simulink model "environment_model_task3"  (Simulink 8.8)
settings: Solver=ode45  StartTime=0.0  StopTime=20000  MaxStep=1  RelTol=1e-3  AbsTol=1e-6  EnableMultiTasking=on
values from neighbouring files (symbols this model uses):
  c = input(5)    [QuatController.m]    (also in main.m = C_optimal; task3b.m = copt)
  k = input(4)    [QuatController.m]    (also in main.m = K_optimal; task3b.m = kopt)
undefined symbols (not defined in the file or in its folder): initial_r, initial_v
settings Model: SuppressorTable=22 serialization::archive 11 0 3 0 0 0 0 0  Creator=menjkim  LastModifiedBy=jamesthomson
settings DataIOCC: SignalLoggingSaveFormat=Dataset  InspectSignalLogs=on
settings OptimizationCC: ExpressionDepthLimit=2147483647
settings DebuggingCC: SolverPrmCheckMsg=warning  FcnCallInpInsideContextMsg=error
settings GRTTargetCC: CombineOutputUpdateFcns=on  GRTInterface=off

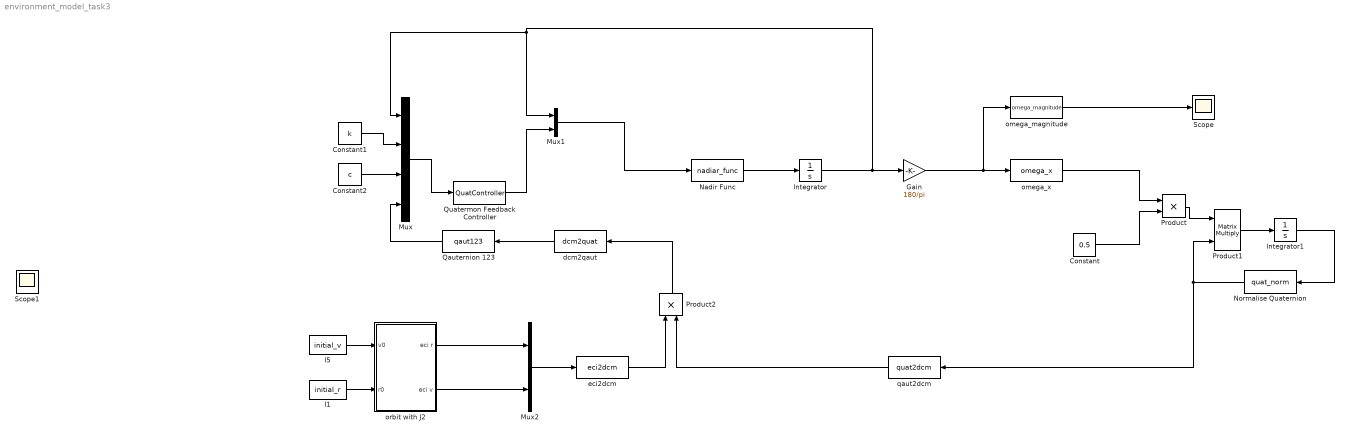
== system environment_model_task3 ==
  Constant : Constant  Value=0.5
  Constant1 : Constant  Value=k
  Constant2 : Constant  Value=c
  Gain : Gain  Gain=180/pi
  I1 : Constant  Value=initial_r
  I5 : Constant  Value=initial_v
  Integrator : Integrator  InitialCondition=[-0.1; 0.1; -0.2]
  Integrator1 : Integrator  InitialCondition=[0.1754; 0.5951; -0.7329; 0.2798]
  Mux : Mux
  Mux1 : Mux  Inputs=2
  Mux2 : Mux  Inputs=2
  Nadir Func : MATLABFcn  MATLABFcn=nadiar_func
  Normalise Quaternion : MATLABFcn  MATLABFcn=quat_norm  Output1D=off
  Product : Product
  Product1 : Product  Multiplication=Matrix(*)
  Product2 : Product
  Qauternion 123 : MATLABFcn  MATLABFcn=qaut123  Output1D=off
  Quatermon Feedback Controller : MATLABFcn  MATLABFcn=QuatController  Output1D=off
  Scope : Scope
  dcm2qaut : MATLABFcn  MATLABFcn=dcm2quat
  eci2dcm : MATLABFcn  MATLABFcn=eci2dcm  Output1D=off
  omega_magnitude : MATLABFcn  MATLABFcn=omega_magnitude
  omega_x : MATLABFcn  MATLABFcn=omega_x  Output1D=off
  orbit with J2 : Subsystem
  qaut2dcm : MATLABFcn  MATLABFcn=quat2dcm  Output1D=off
  Scope1 : Scope
  wires:
  Nadir Func/1 -> Integrator/1
  Integrator/1 -> Mux1/1, Mux/1, Gain/1
  Gain/1 -> omega_magnitude/1, omega_x/1
  omega_x/1 -> Product/1
  Constant/1 -> Product/2
  Product/1 -> Product1/1
  Product1/1 -> Integrator1/1
  omega_magnitude/1 -> Scope/1
  Integrator1/1 -> Normalise Quaternion/1
  I1/1 -> orbit with J2/2(r0)
  I5/1 -> orbit with J2/1(v0)
  eci2dcm/1 -> Product2/1
  Normalise Quaternion/1 -> Product1/2, qaut2dcm/1
  qaut2dcm/1 -> Product2/2
  Product2/1 -> dcm2qaut/1
  dcm2qaut/1 -> Qauternion 123/1
  Mux/1 -> Quatermon Feedback Controller/1
  Quatermon Feedback Controller/1 -> Mux1/2
  Mux1/1 -> Nadir Func/1
  Mux2/1 -> eci2dcm/1
  orbit with J2/1(eci r) -> Mux2/1
  orbit with J2/2(eci v) -> Mux2/2
  Constant1/1 -> Mux/2
  Qauternion 123/1 -> Mux/4
  Constant2/1 -> Mux/3

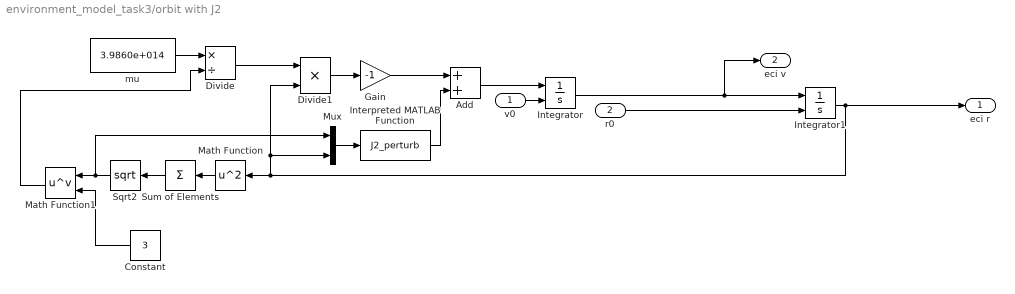
== system environment_model_task3/orbit with J2 ==
  v0 : Inport
  r0 : Inport  Port=2
  Add : Sum
  Constant : Constant  Value=3
  Divide : Product  Inputs=*/
  Divide1 : Product  Inputs=**
  Gain : Gain  Gain=-1
  Integrator : Integrator  InitialConditionSource=external  InitialCondition=[-1021 -88 -7488]
  Integrator1 : Integrator  InitialConditionSource=external  InitialCondition=[596030 -6952400 0]
  Interpreted MATLAB Function : MATLABFcn  MATLABFcn=J2_perturb
  Math Function : Math  Operator=square  SaturateOnIntegerOverflow=on
  Math Function1 : Math  Operator=pow  SaturateOnIntegerOverflow=on
  Mux : Mux  Inputs=2
  Sqrt2 : Math  Operator=sqrt  SaturateOnIntegerOverflow=on
  Sum of Elements : Sum  Inputs=+
  mu : Constant  Value=3.9860e+014
  eci r : Outport
  eci v : Outport  Port=2
  wires:
  r0/1 -> Integrator1/2
  v0/1 -> Integrator/2
  Integrator1/1 -> eci r/1, Math Function/1, Divide1/2, Mux/2
  Sum of Elements/1 -> Sqrt2/1
  Math Function/1 -> Sum of Elements/1
  Divide1/1 -> Gain/1
  Divide/1 -> Divide1/1
  mu/1 -> Divide/1
  Sqrt2/1 -> Mux/1, Math Function1/1
  Math Function1/1 -> Divide/2
  Constant/1 -> Math Function1/2
  Gain/1 -> Add/1
  Add/1 -> Integrator/1
  Mux/1 -> Interpreted MATLAB Function/1
  Interpreted MATLAB Function/1 -> Add/2
  Integrator/1 -> eci v/1, Integrator1/1
